simulink model "pmsm_model"  (R2021a)
settings: Solver=VariableStepAuto  StartTime=0.0  StopTime=10  RelTol=1e-3
values from neighbouring files (symbols this model uses):
  B = 0.01    [pmsm_parameters.m]    (also in test_pmsm.m)
  Cr_ctl_d_D = 0    [pmsm_parameters.m]
  Cr_ctl_d_I = 1    [pmsm_parameters.m]
  Cr_ctl_d_P = 1    [pmsm_parameters.m]
  Cr_ctl_q_D = 0    [pmsm_parameters.m]
  Cr_ctl_q_I = 1    [pmsm_parameters.m]
  Cr_ctl_q_P = 1    [pmsm_parameters.m]
  ctl_mode = 1    [pmsm_parameters.m]
  J_motor = 0.01    [pmsm_parameters.m]    (also in test_pmsm.m)
  L_d = 1.7e-3    (= 0.0017)    [pmsm_parameters.m]    (also in test_pmsm.m)
  L_q = 3.2e-3    (= 0.0032)    [pmsm_parameters.m]    (also in test_pmsm.m)
  lambda = 0.2205    [pmsm_parameters.m]    (also in test_pmsm.m)
  np = 3    [pmsm_parameters.m]    (also in test_pmsm.m)
  Pos_ctl_D = 0    [pmsm_parameters.m]
  Pos_ctl_I = 2    [pmsm_parameters.m]
  Pos_ctl_P = 5    [pmsm_parameters.m]
  R_d = 0.01    [pmsm_parameters.m]    (also in test_pmsm.m)
  R_q = 0.01    [pmsm_parameters.m]    (also in test_pmsm.m)
  Spd_ctl_D = 0    [pmsm_parameters.m]
  Spd_ctl_I = 1    [pmsm_parameters.m]
  Spd_ctl_P = 5    [pmsm_parameters.m]
  Tq_ctl_D = 0    [pmsm_parameters.m]
  Tq_ctl_I = 1    [pmsm_parameters.m]
  Tq_ctl_P = 5    [pmsm_parameters.m]
libraries: pid_lib x5
settings Model: Creator=ge26jow  LastModifiedBy=ge26jow

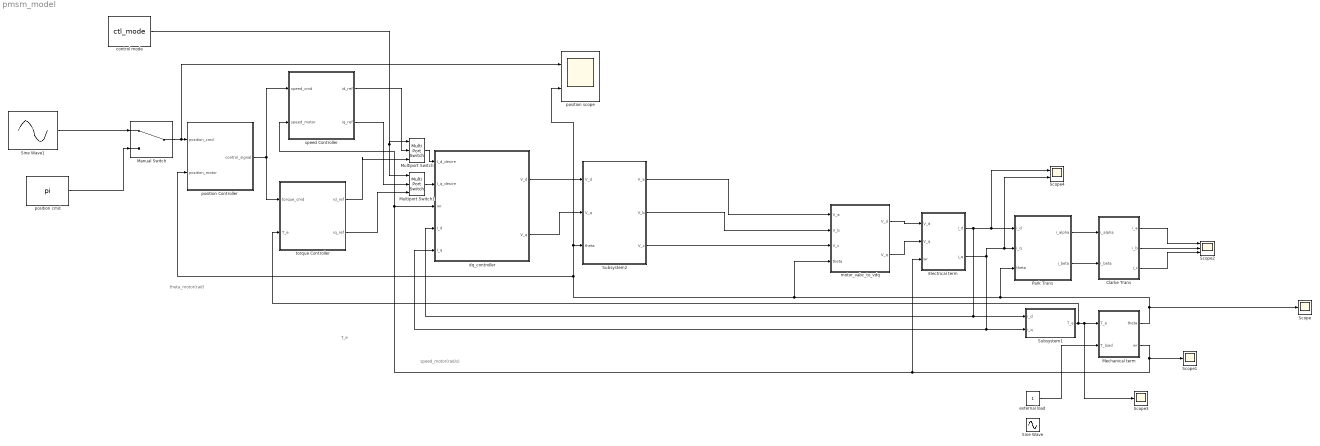
== system pmsm_model ==
  note: speed_motor(rad/s)
  note: T_e
  note: theta_motor(rad)
  Clarke Trans : Subsystem
  Electrical term : Subsystem
  Manual Switch : ManualSwitch
  Mechanical term : Subsystem
  Multiport Switch : MultiPortSwitch  Inputs=2
  Multiport Switch1 : MultiPortSwitch  Inputs=2
  Park Trans : Subsystem
  Scope : Scope
  Scope1 : Scope
  Scope2 : Scope  NumInputPorts=3
  Scope3 : Scope
  Scope4 : Scope  NumInputPorts=2
  Sine Wave : Sin  SampleTime=0
  Sine Wave1 : Sin  SampleTime=0
  Subsystem1 : Subsystem
  Subsystem2 : Subsystem
  control mode : Constant  Value=ctl_mode
  dq_controller : Subsystem
  external load : Constant
  motor_vabc_to_vdq : Subsystem
  position Controller : Subsystem
  position cmd : Constant  Value=pi
  position scope : Scope  NumInputPorts=2
  speed Controller : Subsystem
  torque Controller : Subsystem
  wires:
  Electrical term/1(i_d) -> dq_controller/4(I_d), Subsystem1/1(i_d), Scope4/1, Park Trans/1(i_d)
  Park Trans/1(i_alpha) -> Clarke Trans/1(i_alpha)
  Park Trans/2(i_beta) -> Clarke Trans/2(i_beta)
  Subsystem1/1(T_e) -> torque Controller/2(T_e), Scope3/1, Mechanical term/1(T_e)
  Mechanical term/2(wr) -> Scope1/1, dq_controller/3(wr), speed Controller/2(speed_motor), Electrical term/3(wr)
  Mechanical term/1(theta) -> Scope/1, position Controller/2(position_motor), position scope/2, Subsystem2/3(theta), motor_vabc_to_vdq/4(theta), Park Trans/3(theta)
  external load/1 -> Mechanical term/2(T_load)
  Clarke Trans/1(i_a) -> Scope2/1
  Clarke Trans/2(i_b) -> Scope2/2
  Clarke Trans/3(i_c) -> Scope2/3
  motor_vabc_to_vdq/1(V_d) -> Electrical term/1(V_d)
  motor_vabc_to_vdq/2(V_q) -> Electrical term/2(V_q)
  Electrical term/2(i_q) -> Subsystem1/2(i_q), dq_controller/5(I_q), Scope4/2, Park Trans/2(i_q)
  dq_controller/1(V_d) -> Subsystem2/1(V_d)
  dq_controller/2(V_q) -> Subsystem2/2(V_q)
  Subsystem2/1(V_a) -> motor_vabc_to_vdq/1(V_a)
  Subsystem2/3(V_c) -> motor_vabc_to_vdq/3(V_c)
  Subsystem2/2(V_b) -> motor_vabc_to_vdq/2(V_b)
  position Controller/1(control_signal) -> speed Controller/1(speed_cmd), torque Controller/1(torque_cmd)
  Multiport Switch/1 -> dq_controller/1(I_d_desire)
  Multiport Switch1/1 -> dq_controller/2(I_q_desire)
  torque Controller/2(iq_ref) -> Multiport Switch1/3
  torque Controller/1(id_ref) -> Multiport Switch/3
  speed Controller/2(iq_ref) -> Multiport Switch1/2
  speed Controller/1(id_ref) -> Multiport Switch/2
  control mode/1 -> Multiport Switch1/1, Multiport Switch/1
  Manual Switch/1 -> position scope/1, position Controller/1(position_cmd)
  Sine Wave1/1 -> Manual Switch/1
  position cmd/1 -> Manual Switch/2

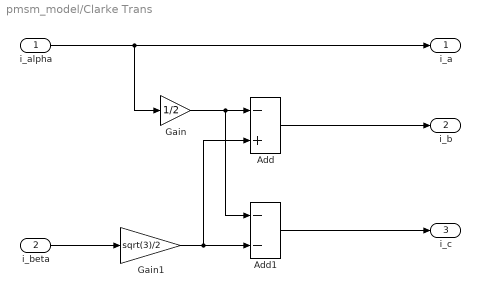
== system pmsm_model/Clarke Trans ==
  i_alpha : Inport
  i_beta : Inport  Port=2
  Add : Sum  Inputs=-+
  Add1 : Sum  Inputs=--
  Gain : Gain  Gain=1/2
  Gain1 : Gain  Gain=sqrt(3)/2
  i_a : Outport
  i_b : Outport  Port=2
  i_c : Outport  Port=3
  wires:
  i_alpha/1 -> Gain/1, i_a/1
  Gain/1 -> Add1/1, Add/1
  i_beta/1 -> Gain1/1
  Gain1/1 -> Add1/2, Add/2
  Add/1 -> i_b/1
  Add1/1 -> i_c/1

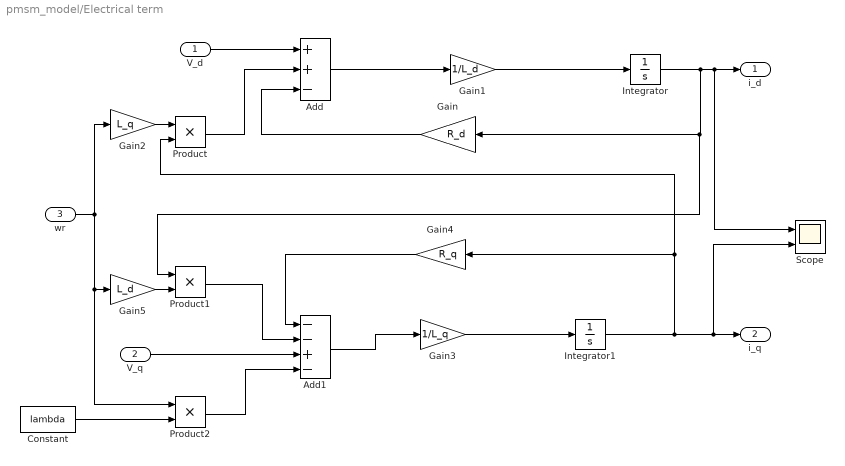
== system pmsm_model/Electrical term ==
  V_d : Inport
  V_q : Inport  Port=2
  wr : Inport  Port=3
  Add : Sum  Inputs=++-
  Add1 : Sum  Inputs=--+-
  Constant : Constant  Value=lambda
  Gain : Gain  Gain=R_d
  Gain1 : Gain  Gain=1/L_d
  Gain2 : Gain  Gain=L_q
  Gain3 : Gain  Gain=1/L_q
  Gain4 : Gain  Gain=R_q
  Gain5 : Gain  Gain=L_d
  Integrator : Integrator
  Integrator1 : Integrator
  Product : Product
  Product1 : Product
  Product2 : Product
  Scope : Scope  NumInputPorts=2
  i_d : Outport
  i_q : Outport  Port=2
  wires:
  V_d/1 -> Add/1
  Add/1 -> Gain1/1
  wr/1 -> Gain2/1, Product2/1, Gain5/1
  Gain2/1 -> Product/1
  Gain1/1 -> Integrator/1
  Product/1 -> Add/2
  Gain/1 -> Add/3
  Integrator/1 -> Product1/1, Gain/1, Scope/1, i_d/1
  Integrator1/1 -> Scope/2, i_q/1, Product/2, Gain4/1
  Add1/1 -> Gain3/1
  Gain3/1 -> Integrator1/1
  Gain4/1 -> Add1/1
  Product1/1 -> Add1/2
  V_q/1 -> Add1/3
  Gain5/1 -> Product1/2
  Constant/1 -> Product2/2
  Product2/1 -> Add1/4

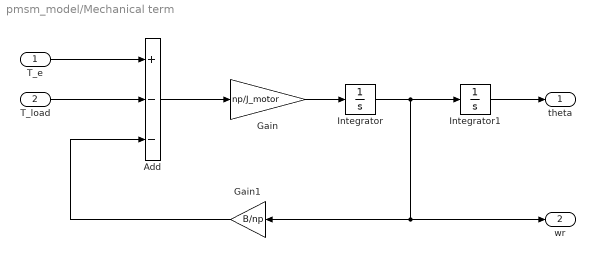
== system pmsm_model/Mechanical term ==
  T_e : Inport
  T_load : Inport  Port=2
  Add : Sum  Inputs=+--
  Gain : Gain  Gain=np/J_motor
  Gain1 : Gain  Gain=B/np
  Integrator : Integrator
  Integrator1 : Integrator
  theta : Outport
  wr : Outport  Port=2
  wires:
  T_e/1 -> Add/1
  T_load/1 -> Add/2
  Add/1 -> Gain/1
  Gain/1 -> Integrator/1
  Gain1/1 -> Add/3
  Integrator/1 -> Gain1/1, wr/1, Integrator1/1
  Integrator1/1 -> theta/1

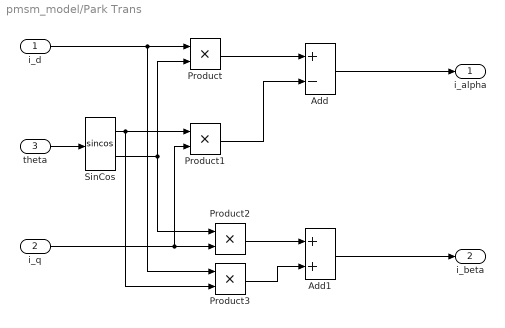
== system pmsm_model/Park Trans ==
  i_d : Inport
  i_q : Inport  Port=2
  theta : Inport  Port=3
  Add : Sum  Inputs=+-
  Add1 : Sum
  Product{,1..3} (4 alike) : Product
  SinCos : Trigonometry  Operator=sincos
  i_alpha : Outport
  i_beta : Outport  Port=2
  wires:
  theta/1 -> SinCos/1
  i_d/1 -> Product3/1, Product/1
  SinCos/2 -> Product2/1, Product/2
  Product/1 -> Add/1
  SinCos/1 -> Product3/2, Product1/1
  i_q/1 -> Product1/2, Product2/2
  Product1/1 -> Add/2
  Add/1 -> i_alpha/1
  Product2/1 -> Add1/1
  Product3/1 -> Add1/2
  Add1/1 -> i_beta/1

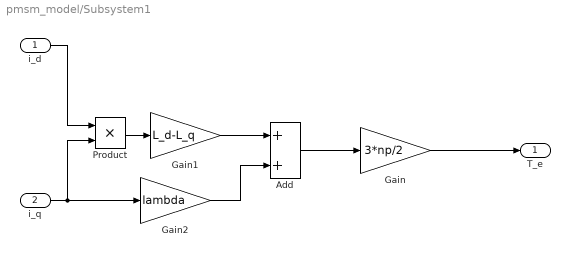
== system pmsm_model/Subsystem1 ==
  i_d : Inport
  i_q : Inport  Port=2
  Add : Sum
  Gain : Gain  Gain=3*np/2
  Gain1 : Gain  Gain=L_d-L_q
  Gain2 : Gain  Gain=lambda
  Product : Product
  T_e : Outport
  wires:
  Add/1 -> Gain/1
  Gain/1 -> T_e/1
  i_q/1 -> Product/2, Gain2/1
  i_d/1 -> Product/1
  Product/1 -> Gain1/1
  Gain1/1 -> Add/1
  Gain2/1 -> Add/2

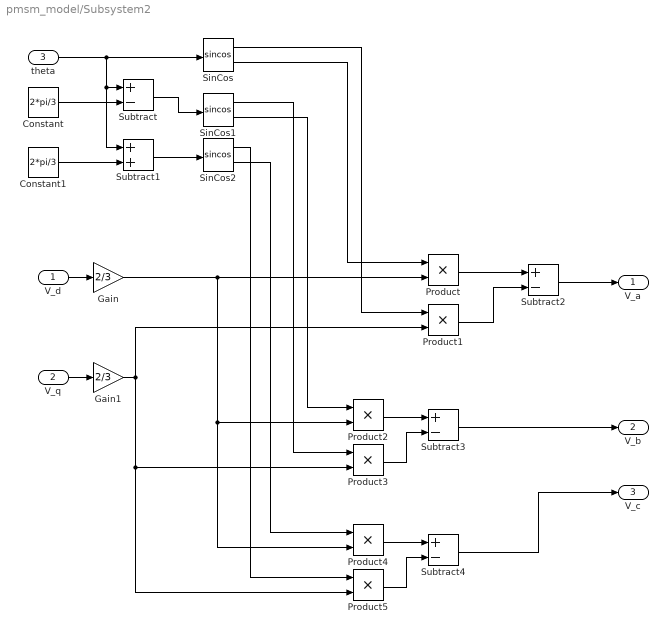
== system pmsm_model/Subsystem2 ==
  V_d : Inport
  V_q : Inport  Port=2
  theta : Inport  Port=3
  Constant : Constant  Value=2*pi/3
  Constant1 : Constant  Value=2*pi/3
  Gain : Gain  Gain=2/3
  Gain1 : Gain  Gain=2/3
  Product{,1..5} (6 alike) : Product
  SinCos : Trigonometry  Operator=sincos
  SinCos1 : Trigonometry  Operator=sincos
  SinCos2 : Trigonometry  Operator=sincos
  Subtract{,2..4} (4 alike) : Sum  Inputs=+-
  Subtract1 : Sum
  V_a : Outport
  V_b : Outport  Port=2
  V_c : Outport  Port=3
  wires:
  Subtract1/1 -> SinCos2/1
  theta/1 -> SinCos/1, Subtract1/1, Subtract/1
  Constant1/1 -> Subtract1/2
  Constant/1 -> Subtract/2
  Subtract/1 -> SinCos1/1
  V_d/1 -> Gain/1
  SinCos/2 -> Product/1
  Product/1 -> Subtract2/1
  Subtract2/1 -> V_a/1
  V_q/1 -> Gain1/1
  SinCos/1 -> Product1/1
  Product1/1 -> Subtract2/2
  SinCos1/2 -> Product2/1
  SinCos1/1 -> Product3/1
  Product2/1 -> Subtract3/1
  Product3/1 -> Subtract3/2
  Subtract3/1 -> V_b/1
  SinCos2/2 -> Product4/1
  SinCos2/1 -> Product5/1
  Product4/1 -> Subtract4/1
  Product5/1 -> Subtract4/2
  Subtract4/1 -> V_c/1
  Gain1/1 -> Product5/2, Product3/2, Product1/2
  Gain/1 -> Product2/2, Product4/2, Product/2

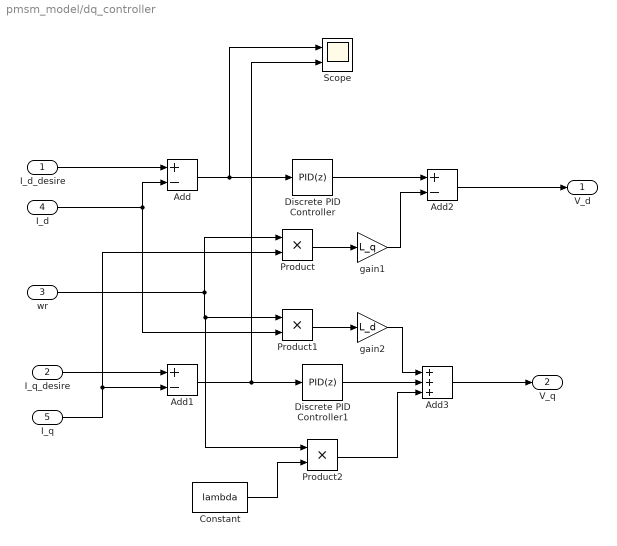
== system pmsm_model/dq_controller ==
  I_d_desire : Inport
  I_q_desire : Inport  Port=2
  wr : Inport  Port=3
  I_d : Inport  Port=4
  I_q : Inport  Port=5
  Add : Sum  Inputs=+-
  Add1 : Sum  Inputs=+-
  Add2 : Sum  Inputs=+-
  Add3 : Sum  Inputs=+++
  Constant : Constant  Value=lambda
  Discrete PID Controller : pid_lib/PID Controller  Controller=PID  Form=Parallel  TimeDomain=Discrete-time  UseExternalTs=off  SampleTime=-1  IntegratorMethod=Forward Euler  FilterMethod=Forward Euler  ControllerParametersSource=internal  P=Cr_ctl_d_P  I=Cr_ctl_d_I  D=Cr_ctl_d_D  UseFilter=on  N=100  TunerSelectOption=Transfer Function Based (PID Tuner App)  InitialConditionSource=internal  InitialConditionForIntegrator=0  InitialConditionForFilter=0  DifferentiatorICPrevScaledInput=0  ExternalReset=none  TrackingMode=off  Kt=1  LimitOutput=off  SatLimitsSource=internal  UpperSaturationLimit=inf  LowerSaturationLimit=-inf  LinearizeAsGain=off  AntiWindupMode=none  Kb=1  POutMin=[]  POutMax=[]  IOutMin=[]  IOutMax=[]  DOutMin=[]  DOutMax=[]  NOutMin=[]  NOutMax=[]  SumOutMin=[]  SumOutMax=[]  SaturationOutMin=[]  SaturationOutMax=[]  PParamMin=[]  PParamMax=[]  IParamMin=[]  IParamMax=[]  DParamMin=[]  DParamMax=[]  NParamMin=[]  NParamMax=[]  KbParamMin=[]  KbParamMax=[]  KtParamMin=[]  KtParamMax=[]  KbOutMin=[]  KbOutMax=[]  KtOutMin=[]  KtOutMax=[]  IntegratorOutMin=[]  IntegratorOutMax=[]  FilterOutMin=[]  FilterOutMax=[]  SumI1OutMin=[]  SumI1OutMax=[]  SumI2OutMin=[]  SumI2OutMax=[]  SumI3OutMin=[]  SumI3OutMax=[]  SumI4OutMin=[]  SumI4OutMax=[]  SumDOutMin=[]  SumDOutMax=[]  DifferentiatorOutMin=[]  DifferentiatorOutMax=[]  FilterDiffOutCoefMin=[]  FilterDiffOutCoefMax=[]  ReciprocalOutMin=[]  ReciprocalOutMax=[]  SumDenOutMin=[]  SumDenOutMax=[]  SumNumOutMin=[]  SumNumOutMax=[]  DivideOutMin=[]  DivideOutMax=[]  UdiffTsProdOutMin=[]  UdiffTsProdOutMax=[]  NTsProdOutMin=[]  NTsProdOutMax=[]  UintegralTsProdOutMin=[]  UintegralTsProdOutMax=[]  UngainTsProdOutMin=[]  UngainTsProdOutMax=[]  IntegratorContinuousStateAttributes=''  IntegratorStateMustResolveToSignalObject=off  IntegratorRTWStateStorageClass=Auto  FilterContinuousStateAttributes=''  FilterStateMustResolveToSignalObject=off  FilterRTWStateStorageClass=Auto  ParallelPVariant=InternalParameters  IdealPVariant=Disabled  IVariant=InternalParameters  DVariant=InternalParameters  IntegratorVariant=Discrete  SatVariant=Disabled  AWVariant=Passthrough  PCopyVariant=Disabled  TRVariant=Disabled  FdbkBlocksVariant=Forward  IdealPFdbkVariant=Disabled  SatFdbkVariant=Disabled  DerivativeFilterVariant=ForwardEulerFilter  NVariant=InternalParameters  NCopyVariant=Disabled  FilterICVariant=InternalICsFilter  IntegratorICVariant=InternalICs  ExternalResetVariant=Disabled  TRSumVariant=Passthrough  SumFdbkVariant=Disabled  SumVariant=Sum_PID  TsampFilterVariant=InternalTs  TsampNgainVariant=Passthrough  TsampIntegralVariant=Passthrough  ExternalSaturationOutDataTypeStr=Inherit: Same as second input
  Discrete PID Controller1 : pid_lib/PID Controller  Controller=PID  Form=Parallel  TimeDomain=Discrete-time  UseExternalTs=off  SampleTime=-1  IntegratorMethod=Forward Euler  FilterMethod=Forward Euler  ControllerParametersSource=internal  P=Cr_ctl_q_P  I=Cr_ctl_q_I  D=Cr_ctl_q_D  UseFilter=on  N=100  TunerSelectOption=Transfer Function Based (PID Tuner App)  InitialConditionSource=internal  InitialConditionForIntegrator=0  InitialConditionForFilter=0  DifferentiatorICPrevScaledInput=0  ExternalReset=none  TrackingMode=off  Kt=1  LimitOutput=off  SatLimitsSource=internal  UpperSaturationLimit=inf  LowerSaturationLimit=-inf  LinearizeAsGain=off  AntiWindupMode=none  Kb=1  POutMin=[]  POutMax=[]  IOutMin=[]  IOutMax=[]  DOutMin=[]  DOutMax=[]  NOutMin=[]  NOutMax=[]  SumOutMin=[]  SumOutMax=[]  SaturationOutMin=[]  SaturationOutMax=[]  PParamMin=[]  PParamMax=[]  IParamMin=[]  IParamMax=[]  DParamMin=[]  DParamMax=[]  NParamMin=[]  NParamMax=[]  KbParamMin=[]  KbParamMax=[]  KtParamMin=[]  KtParamMax=[]  KbOutMin=[]  KbOutMax=[]  KtOutMin=[]  KtOutMax=[]  IntegratorOutMin=[]  IntegratorOutMax=[]  FilterOutMin=[]  FilterOutMax=[]  SumI1OutMin=[]  SumI1OutMax=[]  SumI2OutMin=[]  SumI2OutMax=[]  SumI3OutMin=[]  SumI3OutMax=[]  SumI4OutMin=[]  SumI4OutMax=[]  SumDOutMin=[]  SumDOutMax=[]  DifferentiatorOutMin=[]  DifferentiatorOutMax=[]  FilterDiffOutCoefMin=[]  FilterDiffOutCoefMax=[]  ReciprocalOutMin=[]  ReciprocalOutMax=[]  SumDenOutMin=[]  SumDenOutMax=[]  SumNumOutMin=[]  SumNumOutMax=[]  DivideOutMin=[]  DivideOutMax=[]  UdiffTsProdOutMin=[]  UdiffTsProdOutMax=[]  NTsProdOutMin=[]  NTsProdOutMax=[]  UintegralTsProdOutMin=[]  UintegralTsProdOutMax=[]  UngainTsProdOutMin=[]  UngainTsProdOutMax=[]  IntegratorContinuousStateAttributes=''  IntegratorStateMustResolveToSignalObject=off  IntegratorRTWStateStorageClass=Auto  FilterContinuousStateAttributes=''  FilterStateMustResolveToSignalObject=off  FilterRTWStateStorageClass=Auto  ParallelPVariant=InternalParameters  IdealPVariant=Disabled  IVariant=InternalParameters  DVariant=InternalParameters  IntegratorVariant=Discrete  SatVariant=Disabled  AWVariant=Passthrough  PCopyVariant=Disabled  TRVariant=Disabled  FdbkBlocksVariant=Forward  IdealPFdbkVariant=Disabled  SatFdbkVariant=Disabled  DerivativeFilterVariant=ForwardEulerFilter  NVariant=InternalParameters  NCopyVariant=Disabled  FilterICVariant=InternalICsFilter  IntegratorICVariant=InternalICs  ExternalResetVariant=Disabled  TRSumVariant=Passthrough  SumFdbkVariant=Disabled  SumVariant=Sum_PID  TsampFilterVariant=InternalTs  TsampNgainVariant=Passthrough  TsampIntegralVariant=Passthrough  ExternalSaturationOutDataTypeStr=Inherit: Same as second input
  Product : Product
  Product1 : Product
  Product2 : Product
  Scope : Scope  NumInputPorts=2
  gain1 : Gain  Gain=L_q
  gain2 : Gain  Gain=L_d
  V_d : Outport
  V_q : Outport  Port=2
  wires:
  I_d_desire/1 -> Add/1
  I_d/1 -> Product1/2, Add/2
  I_q_desire/1 -> Add1/1
  I_q/1 -> Add1/2, Product/2
  Add/1 -> Scope/1, Discrete PID Controller/1
  wr/1 -> Product2/1, Product1/1, Product/1
  Product/1 -> gain1/1
  Discrete PID Controller/1 -> Add2/1
  Add1/1 -> Scope/2, Discrete PID Controller1/1
  gain1/1 -> Add2/2
  Add2/1 -> V_d/1
  Product1/1 -> gain2/1
  Discrete PID Controller1/1 -> Add3/2
  gain2/1 -> Add3/1
  Add3/1 -> V_q/1
  Constant/1 -> Product2/2
  Product2/1 -> Add3/3

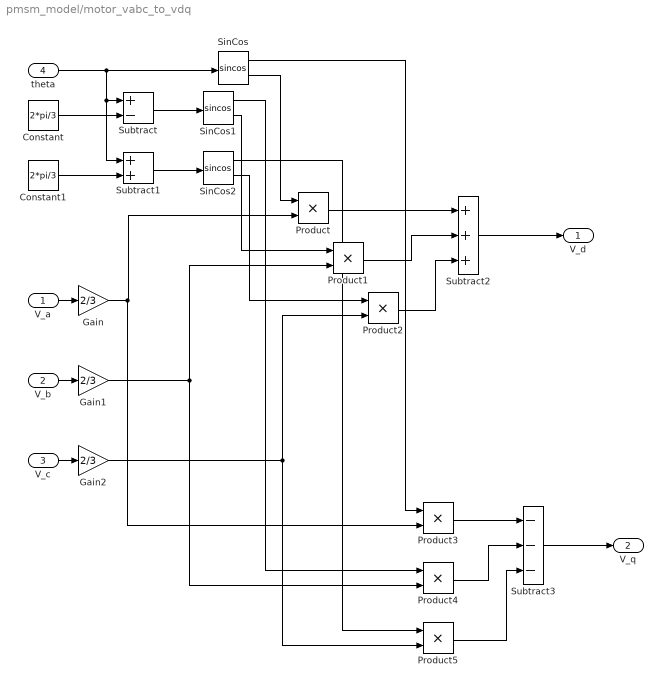
== system pmsm_model/motor_vabc_to_vdq ==
  V_a : Inport
  V_b : Inport  Port=2
  V_c : Inport  Port=3
  theta : Inport  Port=4
  Constant : Constant  Value=2*pi/3
  Constant1 : Constant  Value=2*pi/3
  Gain : Gain  Gain=2/3
  Gain1 : Gain  Gain=2/3
  Gain2 : Gain  Gain=2/3
  Product{,1..5} (6 alike) : Product
  SinCos : Trigonometry  Operator=sincos
  SinCos1 : Trigonometry  Operator=sincos
  SinCos2 : Trigonometry  Operator=sincos
  Subtract : Sum  Inputs=+-
  Subtract1 : Sum
  Subtract2 : Sum  Inputs=+++
  Subtract3 : Sum  Inputs=---
  V_d : Outport
  V_q : Outport  Port=2
  wires:
  theta/1 -> SinCos/1, Subtract1/1, Subtract/1
  V_a/1 -> Gain/1
  SinCos/2 -> Product/1
  Constant/1 -> Subtract/2
  Subtract/1 -> SinCos1/1
  V_b/1 -> Gain1/1
  SinCos1/2 -> Product1/1
  Subtract1/1 -> SinCos2/1
  Constant1/1 -> Subtract1/2
  V_c/1 -> Gain2/1
  SinCos2/2 -> Product2/1
  Product/1 -> Subtract2/1
  Product1/1 -> Subtract2/2
  Product2/1 -> Subtract2/3
  Subtract2/1 -> V_d/1
  SinCos/1 -> Product3/1
  SinCos1/1 -> Product4/1
  SinCos2/1 -> Product5/1
  Product3/1 -> Subtract3/1
  Product4/1 -> Subtract3/2
  Product5/1 -> Subtract3/3
  Subtract3/1 -> V_q/1
  Gain1/1 -> Product4/2, Product1/2
  Gain/1 -> Product3/2, Product/2
  Gain2/1 -> Product5/2, Product2/2

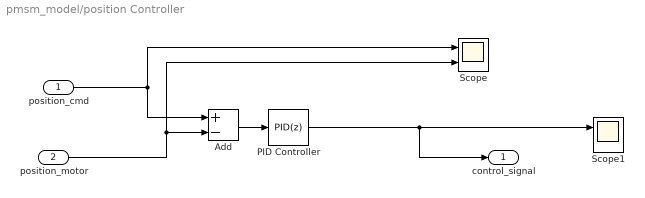
== system pmsm_model/position Controller ==
  position_cmd : Inport  SampleTime=1e-3
  position_motor : Inport  Port=2  SampleTime=1e-3
  Add : Sum  Inputs=+-
  PID Controller : pid_lib/PID Controller  Controller=PID  Form=Parallel  TimeDomain=Discrete-time  UseExternalTs=off  SampleTime=-1  IntegratorMethod=Forward Euler  FilterMethod=Forward Euler  ControllerParametersSource=internal  P=Pos_ctl_P  I=Pos_ctl_I  D=Pos_ctl_D  UseFilter=on  N=100  TunerSelectOption=Transfer Function Based (PID Tuner App)  InitialConditionSource=internal  InitialConditionForIntegrator=0  InitialConditionForFilter=0  DifferentiatorICPrevScaledInput=0  ExternalReset=none  TrackingMode=off  Kt=1  LimitOutput=off  SatLimitsSource=internal  UpperSaturationLimit=inf  LowerSaturationLimit=-inf  LinearizeAsGain=on  AntiWindupMode=none  Kb=1  POutMin=[]  POutMax=[]  IOutMin=[]  IOutMax=[]  DOutMin=[]  DOutMax=[]  NOutMin=[]  NOutMax=[]  SumOutMin=[]  SumOutMax=[]  SaturationOutMin=[]  SaturationOutMax=[]  PParamMin=[]  PParamMax=[]  IParamMin=[]  IParamMax=[]  DParamMin=[]  DParamMax=[]  NParamMin=[]  NParamMax=[]  KbParamMin=[]  KbParamMax=[]  KtParamMin=[]  KtParamMax=[]  KbOutMin=[]  KbOutMax=[]  KtOutMin=[]  KtOutMax=[]  IntegratorOutMin=[]  IntegratorOutMax=[]  FilterOutMin=[]  FilterOutMax=[]  SumI1OutMin=[]  SumI1OutMax=[]  SumI2OutMin=[]  SumI2OutMax=[]  SumI3OutMin=[]  SumI3OutMax=[]  SumI4OutMin=[]  SumI4OutMax=[]  SumDOutMin=[]  SumDOutMax=[]  DifferentiatorOutMin=[]  DifferentiatorOutMax=[]  FilterDiffOutCoefMin=[]  FilterDiffOutCoefMax=[]  ReciprocalOutMin=[]  ReciprocalOutMax=[]  SumDenOutMin=[]  SumDenOutMax=[]  SumNumOutMin=[]  SumNumOutMax=[]  DivideOutMin=[]  DivideOutMax=[]  UdiffTsProdOutMin=[]  UdiffTsProdOutMax=[]  NTsProdOutMin=[]  NTsProdOutMax=[]  UintegralTsProdOutMin=[]  UintegralTsProdOutMax=[]  UngainTsProdOutMin=[]  UngainTsProdOutMax=[]  IntegratorContinuousStateAttributes=''  IntegratorStateMustResolveToSignalObject=off  IntegratorRTWStateStorageClass=Auto  FilterContinuousStateAttributes=''  FilterStateMustResolveToSignalObject=off  FilterRTWStateStorageClass=Auto  ParallelPVariant=InternalParameters  IdealPVariant=Disabled  IVariant=InternalParameters  DVariant=InternalParameters  IntegratorVariant=Discrete  SatVariant=Disabled  AWVariant=Passthrough  PCopyVariant=Disabled  TRVariant=Disabled  FdbkBlocksVariant=Forward  IdealPFdbkVariant=Disabled  SatFdbkVariant=Disabled  DerivativeFilterVariant=ForwardEulerFilter  NVariant=InternalParameters  NCopyVariant=Disabled  FilterICVariant=InternalICsFilter  IntegratorICVariant=InternalICs  ExternalResetVariant=Disabled  TRSumVariant=Passthrough  SumFdbkVariant=Disabled  SumVariant=Sum_PID  TsampFilterVariant=InternalTs  TsampNgainVariant=Passthrough  TsampIntegralVariant=Passthrough  ExternalSaturationOutDataTypeStr=Inherit: Same as second input
  Scope : Scope  NumInputPorts=2
  Scope1 : Scope  NumInputPorts=2
  control_signal : Outport  VectorParamsAs1DForOutWhenUnconnected=off
  wires:
  PID Controller/1 -> control_signal/1, Scope1/1
  Add/1 -> PID Controller/1
  position_cmd/1 -> Scope/1, Add/1
  position_motor/1 -> Scope/2, Add/2

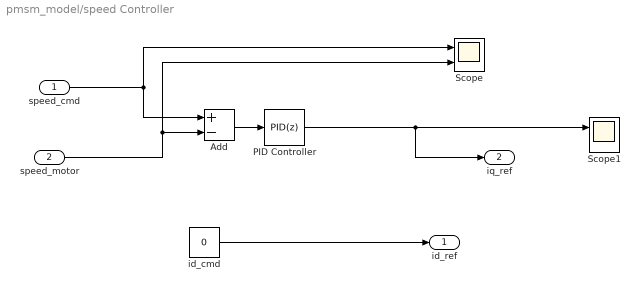
== system pmsm_model/speed Controller ==
  speed_cmd : Inport  SampleTime=1e-3
  speed_motor : Inport  Port=2  SampleTime=1e-3
  Add : Sum  Inputs=+-
  PID Controller : pid_lib/PID Controller  Controller=PID  Form=Parallel  TimeDomain=Discrete-time  UseExternalTs=off  SampleTime=-1  IntegratorMethod=Forward Euler  FilterMethod=Forward Euler  ControllerParametersSource=internal  P=Spd_ctl_P  I=Spd_ctl_I  D=Spd_ctl_D  UseFilter=on  N=100  TunerSelectOption=Transfer Function Based (PID Tuner App)  InitialConditionSource=internal  InitialConditionForIntegrator=0  InitialConditionForFilter=0  DifferentiatorICPrevScaledInput=0  ExternalReset=none  TrackingMode=off  Kt=1  LimitOutput=off  SatLimitsSource=internal  UpperSaturationLimit=inf  LowerSaturationLimit=-inf  LinearizeAsGain=on  AntiWindupMode=none  Kb=1  POutMin=[]  POutMax=[]  IOutMin=[]  IOutMax=[]  DOutMin=[]  DOutMax=[]  NOutMin=[]  NOutMax=[]  SumOutMin=[]  SumOutMax=[]  SaturationOutMin=[]  SaturationOutMax=[]  PParamMin=[]  PParamMax=[]  IParamMin=[]  IParamMax=[]  DParamMin=[]  DParamMax=[]  NParamMin=[]  NParamMax=[]  KbParamMin=[]  KbParamMax=[]  KtParamMin=[]  KtParamMax=[]  KbOutMin=[]  KbOutMax=[]  KtOutMin=[]  KtOutMax=[]  IntegratorOutMin=[]  IntegratorOutMax=[]  FilterOutMin=[]  FilterOutMax=[]  SumI1OutMin=[]  SumI1OutMax=[]  SumI2OutMin=[]  SumI2OutMax=[]  SumI3OutMin=[]  SumI3OutMax=[]  SumI4OutMin=[]  SumI4OutMax=[]  SumDOutMin=[]  SumDOutMax=[]  DifferentiatorOutMin=[]  DifferentiatorOutMax=[]  FilterDiffOutCoefMin=[]  FilterDiffOutCoefMax=[]  ReciprocalOutMin=[]  ReciprocalOutMax=[]  SumDenOutMin=[]  SumDenOutMax=[]  SumNumOutMin=[]  SumNumOutMax=[]  DivideOutMin=[]  DivideOutMax=[]  UdiffTsProdOutMin=[]  UdiffTsProdOutMax=[]  NTsProdOutMin=[]  NTsProdOutMax=[]  UintegralTsProdOutMin=[]  UintegralTsProdOutMax=[]  UngainTsProdOutMin=[]  UngainTsProdOutMax=[]  IntegratorContinuousStateAttributes=''  IntegratorStateMustResolveToSignalObject=off  IntegratorRTWStateStorageClass=Auto  FilterContinuousStateAttributes=''  FilterStateMustResolveToSignalObject=off  FilterRTWStateStorageClass=Auto  ParallelPVariant=InternalParameters  IdealPVariant=Disabled  IVariant=InternalParameters  DVariant=InternalParameters  IntegratorVariant=Discrete  SatVariant=Disabled  AWVariant=Passthrough  PCopyVariant=Disabled  TRVariant=Disabled  FdbkBlocksVariant=Forward  IdealPFdbkVariant=Disabled  SatFdbkVariant=Disabled  DerivativeFilterVariant=ForwardEulerFilter  NVariant=InternalParameters  NCopyVariant=Disabled  FilterICVariant=InternalICsFilter  IntegratorICVariant=InternalICs  ExternalResetVariant=Disabled  TRSumVariant=Passthrough  SumFdbkVariant=Disabled  SumVariant=Sum_PID  TsampFilterVariant=InternalTs  TsampNgainVariant=Passthrough  TsampIntegralVariant=Passthrough  ExternalSaturationOutDataTypeStr=Inherit: Same as second input
  Scope : Scope  NumInputPorts=2
  Scope1 : Scope  NumInputPorts=2
  id_cmd : Constant  Value=0  SampleTime=1e-3
  id_ref : Outport  VectorParamsAs1DForOutWhenUnconnected=off
  iq_ref : Outport  Port=2  VectorParamsAs1DForOutWhenUnconnected=off
  wires:
  id_cmd/1 -> id_ref/1
  PID Controller/1 -> iq_ref/1, Scope1/1
  Add/1 -> PID Controller/1
  speed_cmd/1 -> Scope/1, Add/1
  speed_motor/1 -> Scope/2, Add/2

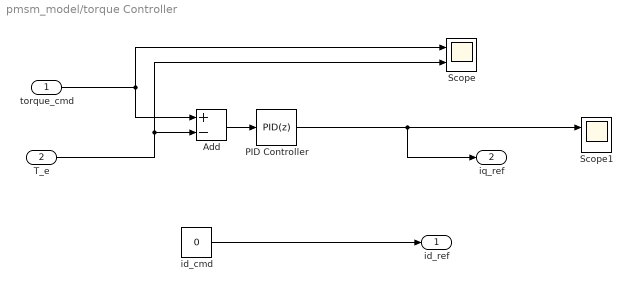
== system pmsm_model/torque Controller ==
  torque_cmd : Inport  SampleTime=1e-3
  T_e : Inport  Port=2  SampleTime=1e-3
  Add : Sum  Inputs=+-
  PID Controller : pid_lib/PID Controller  Controller=PID  Form=Parallel  TimeDomain=Discrete-time  UseExternalTs=off  SampleTime=-1  IntegratorMethod=Forward Euler  FilterMethod=Forward Euler  ControllerParametersSource=internal  P=Tq_ctl_P  I=Tq_ctl_I  D=Tq_ctl_D  UseFilter=on  N=100  TunerSelectOption=Transfer Function Based (PID Tuner App)  InitialConditionSource=internal  InitialConditionForIntegrator=0  InitialConditionForFilter=0  DifferentiatorICPrevScaledInput=0  ExternalReset=none  TrackingMode=off  Kt=1  LimitOutput=off  SatLimitsSource=internal  UpperSaturationLimit=inf  LowerSaturationLimit=-inf  LinearizeAsGain=on  AntiWindupMode=none  Kb=1  POutMin=[]  POutMax=[]  IOutMin=[]  IOutMax=[]  DOutMin=[]  DOutMax=[]  NOutMin=[]  NOutMax=[]  SumOutMin=[]  SumOutMax=[]  SaturationOutMin=[]  SaturationOutMax=[]  PParamMin=[]  PParamMax=[]  IParamMin=[]  IParamMax=[]  DParamMin=[]  DParamMax=[]  NParamMin=[]  NParamMax=[]  KbParamMin=[]  KbParamMax=[]  KtParamMin=[]  KtParamMax=[]  KbOutMin=[]  KbOutMax=[]  KtOutMin=[]  KtOutMax=[]  IntegratorOutMin=[]  IntegratorOutMax=[]  FilterOutMin=[]  FilterOutMax=[]  SumI1OutMin=[]  SumI1OutMax=[]  SumI2OutMin=[]  SumI2OutMax=[]  SumI3OutMin=[]  SumI3OutMax=[]  SumI4OutMin=[]  SumI4OutMax=[]  SumDOutMin=[]  SumDOutMax=[]  DifferentiatorOutMin=[]  DifferentiatorOutMax=[]  FilterDiffOutCoefMin=[]  FilterDiffOutCoefMax=[]  ReciprocalOutMin=[]  ReciprocalOutMax=[]  SumDenOutMin=[]  SumDenOutMax=[]  SumNumOutMin=[]  SumNumOutMax=[]  DivideOutMin=[]  DivideOutMax=[]  UdiffTsProdOutMin=[]  UdiffTsProdOutMax=[]  NTsProdOutMin=[]  NTsProdOutMax=[]  UintegralTsProdOutMin=[]  UintegralTsProdOutMax=[]  UngainTsProdOutMin=[]  UngainTsProdOutMax=[]  IntegratorContinuousStateAttributes=''  IntegratorStateMustResolveToSignalObject=off  IntegratorRTWStateStorageClass=Auto  FilterContinuousStateAttributes=''  FilterStateMustResolveToSignalObject=off  FilterRTWStateStorageClass=Auto  ParallelPVariant=InternalParameters  IdealPVariant=Disabled  IVariant=InternalParameters  DVariant=InternalParameters  IntegratorVariant=Discrete  SatVariant=Disabled  AWVariant=Passthrough  PCopyVariant=Disabled  TRVariant=Disabled  FdbkBlocksVariant=Forward  IdealPFdbkVariant=Disabled  SatFdbkVariant=Disabled  DerivativeFilterVariant=ForwardEulerFilter  NVariant=InternalParameters  NCopyVariant=Disabled  FilterICVariant=InternalICsFilter  IntegratorICVariant=InternalICs  ExternalResetVariant=Disabled  TRSumVariant=Passthrough  SumFdbkVariant=Disabled  SumVariant=Sum_PID  TsampFilterVariant=InternalTs  TsampNgainVariant=Passthrough  TsampIntegralVariant=Passthrough  ExternalSaturationOutDataTypeStr=Inherit: Same as second input
  Scope : Scope  NumInputPorts=2
  Scope1 : Scope  NumInputPorts=2
  id_cmd : Constant  Value=0  SampleTime=1e-3
  id_ref : Outport  VectorParamsAs1DForOutWhenUnconnected=off
  iq_ref : Outport  Port=2  VectorParamsAs1DForOutWhenUnconnected=off
  wires:
  id_cmd/1 -> id_ref/1
  PID Controller/1 -> iq_ref/1, Scope1/1
  Add/1 -> PID Controller/1
  torque_cmd/1 -> Scope/1, Add/1
  T_e/1 -> Scope/2, Add/2
